simulink model "CNcs7"  (Simulink 6.2)
settings: Solver=ode4  SolverMode=SingleTasking  StartTime=0.0  StopTime=5  FixedStep=0.001  MaxStep=0.001  RelTol=1e-3  AbsTol=1e-3
undefined symbols (not defined in the file): alexlaw, bs_onoff, bs_scale, bsfsacrit, bsfsvcrit, cnsgain, fs_onoff, fs_scale, fsdelaycalc, ltdrk, phasicgain, pmcgain, pmctau2, pmctau3, saccrefract, saccsw, spgain, tonicgain, tvrD, tvrN, velnoise, velreconsw
libraries: simulink_extras x38, simulink x2
(part 2 of 5)

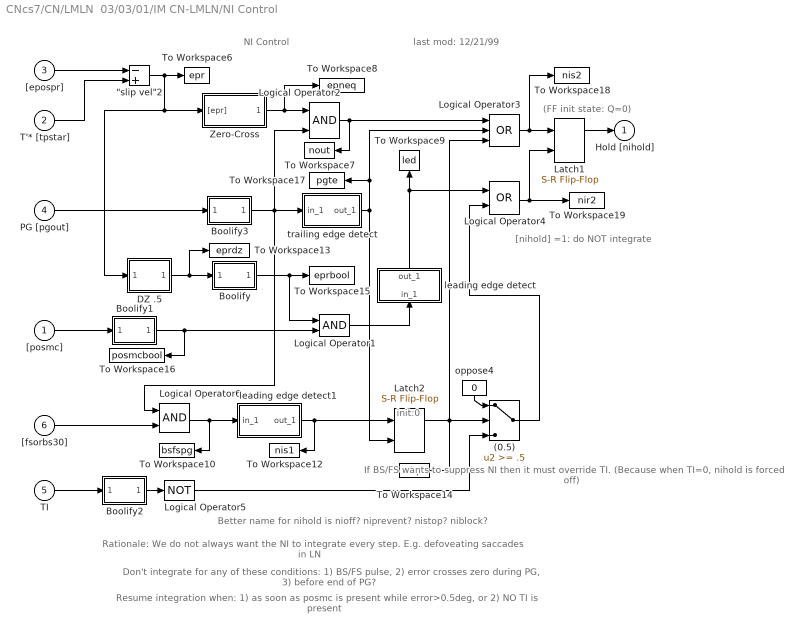
== system CNcs7/CN/LMLN  03/03/01/IM CN-LMLN/NI Control ==
  note: (FF init state: Q=0)
  note: NI Control
  note: If BS/FS wants to suppress NI
      | then it must override TI. (Because
      | when TI=0, nihold is forced off)
  note: last mod:
      | 12/21/99
  note: Rationale: We do not always want the NI to integrate every step. E.g. defoveating saccades in LN
  note: Don't integrate for any of these conditions: 1) BS/FS pulse, 2) error crosses zero during PG, 3) before end of PG?
  note: [nihold] =1: do NOT integrate
  note: init:0
  note: Better name for nihold is nioff? niprevent? nistop? niblock?
  note: Resume integration when: 1) as soon as posmc is present while error>0.5deg, or 2) NO TI is present
  "[posmc]" : Inport  Port=1  LatchInput=off
  T'* [tpstar] : Inport  Port=2  LatchInput=off
  "[epospr]" : Inport  Port=3  LatchInput=off
  PG [pgout] : Inport  Port=4  LatchInput=off
  TI : Inport  Port=5  LatchInput=off
  "[fsorbs30]" : Inport  Port=6  LatchInput=off
  "\"slip vel\"2" : Sum  Inputs=-+  SaturateOnIntegerOverflow=on  InputSameDT=on
  (0.5) : Switch  Threshold=.5  SaturateOnIntegerOverflow=on  InputSameDT=on
  Boolify : Subsystem
      mask Display: disp('Boolify')
  Boolify1 : Subsystem
      mask Display: disp('Boolify')
  Boolify2 : Subsystem
      mask Display: disp('Boolify')
  Boolify3 : Subsystem
      mask Display: disp('Boolify')
  DZ .5 : Subsystem
      mask Display: disp('Dead\nZone')
  Latch1 : simulink_extras/Flip Flops/S-R Flip-Flop  initial_condition=0
  Latch2 : simulink_extras/Flip Flops/S-R Flip-Flop  initial_condition=0
  Logical Operator1 : Logic
  Logical Operator2 : Logic
  Logical Operator3 : Logic  Operator=OR  Inputs=3
  Logical Operator4 : Logic  Operator=OR
  Logical Operator5 : Logic  Operator=NOT  Inputs=1
  Logical Operator6 : Logic
  To Workspace10 : ToWorkspace  VariableName=bsfspg  SaveFormat=Array
      settings: MaxDataPoints=10000
  To Workspace12 : ToWorkspace  VariableName=nis1  SaveFormat=Array
      settings: MaxDataPoints=10000
  To Workspace13 : ToWorkspace  VariableName=eprdz  SaveFormat=Array
      settings: MaxDataPoints=10000
  To Workspace14 : ToWorkspace  VariableName=niq1  SaveFormat=Array
      settings: MaxDataPoints=10000
  To Workspace15 : ToWorkspace  VariableName=eprbool  SaveFormat=Array
      settings: MaxDataPoints=10000
  To Workspace16 : ToWorkspace  VariableName=posmcbool  SaveFormat=Array
      settings: MaxDataPoints=10000
  To Workspace17 : ToWorkspace  VariableName=pgte  SaveFormat=Array
      settings: MaxDataPoints=10000
  To Workspace18 : ToWorkspace  VariableName=nis2  SaveFormat=Array
      settings: MaxDataPoints=10000
  To Workspace19 : ToWorkspace  VariableName=nir2  SaveFormat=Array
      settings: MaxDataPoints=10000
  To Workspace6 : ToWorkspace  VariableName=epr  SaveFormat=Array
      settings: MaxDataPoints=10000
  To Workspace7 : ToWorkspace  VariableName=nout  SaveFormat=Array
      settings: MaxDataPoints=10000
  To Workspace8 : ToWorkspace  VariableName=epneq  SaveFormat=Array
      settings: MaxDataPoints=10000
  To Workspace9 : ToWorkspace  VariableName=led  SaveFormat=Array
      settings: Orientation=up  MaxDataPoints=10000
  Zero-Cross : Subsystem
      mask Display: disp('Zero-Cross\nDetect')
  leading edge detect : Subsystem  Orientation=up
      mask Display: disp('Leading\nEdge Det')
  leading edge detect1 : Subsystem
      mask Display: disp('Leading\nEdge Det')
  oppose4 : Constant  Orientation=down  Value=0
  trailing edge detect : Subsystem
      mask Display: disp('Trailing\nEdge Det')
  Hold [nihold] : Outport
  wires:
  T'* [tpstar]/1 -> "\"slip vel\"2"/2
  PG [pgout]/1 -> Boolify3/1(In1)
  "\"slip vel\"2"/1 -> To Workspace6/1, DZ .5/1(in_1), Zero-Cross/1("[epr]")
  "[epospr]"/1 -> "\"slip vel\"2"/1
  Latch1/1 -> Hold [nihold]/1
  Logical Operator3/1 -> Latch1/1, To Workspace18/1
  Zero-Cross/1("[epneq]") -> Logical Operator2/1, To Workspace8/1
  Logical Operator1/1 -> leading edge detect/1(in_1)
  Logical Operator2/1 -> Logical Operator3/1, To Workspace7/1
  "[fsorbs30]"/1 -> Logical Operator6/2
  Logical Operator6/1 -> leading edge detect1/1(in_1), To Workspace10/1
  Latch2/1 -> Logical Operator3/3, (0.5)/2, To Workspace14/1
  oppose4/1 -> (0.5)/1
  Logical Operator5/1 -> (0.5)/3
  leading edge detect1/1(out_1) -> Latch2/1, To Workspace12/1
  Logical Operator4/1 -> Latch1/2, To Workspace19/1
  TI/1 -> Boolify2/1(In1)
  Boolify2/1(Out1) -> Logical Operator5/1
  leading edge detect/1(out_1) -> To Workspace9/1, Logical Operator4/1
  (0.5)/1 -> Logical Operator4/2
  Boolify3/1(Out1) -> Logical Operator6/1, trailing edge detect/1(in_1), Logical Operator2/2
  trailing edge detect/1(out_1) -> To Workspace17/1, Logical Operator3/2, Latch2/2
  Boolify/1(Out1) -> To Workspace15/1, Logical Operator1/1
  DZ .5/1(out_1) -> Boolify/1(In1), To Workspace13/1
  "[posmc]"/1 -> Boolify1/1(In1)
  Boolify1/1(Out1) -> To Workspace16/1, Logical Operator1/2

== system CNcs7/CN/LMLN  03/03/01/IM CN-LMLN/Sacc Blank ==
  note: Saccade and Post-Saccadic Drift Blanking
  note: (FF init state: Q=1)
  note: "Is RetVel Err increaing?"
  note: really an "enable"
      | signal?
  note: last mod:
      | 02/03/00
  note: [sbsac]  is initially ENABLED, and is DISABLED by  the leading edge of a saccade
      |  (after an 80ms delay).  70 ms later the timer REENABLES [sbsac]
      | (Because of the 80ms delay, actual time of reenable is150 ms after end of PG)
  note: Lower SR latch is SET by [sbsac] going high.  The switch will now pass information
      | about the change in velocity error (whether it is decreasing or increasing).
      | If it is increasing, [sbsp] is 1, and the beginning of this increase sets the switch so
      | that [sbsp] = [sbsac].  If the error is decreasing, then [sbsp] = 0, and should stay 0
      |  for as long as [velerr] is decreasing ***and hasn't crossed zero***
  note: Rationale: We do not want the model to look at the slow phase information that immediately
      | follows a saccade.   We want to disable both the saccadic and SP systems appropriately.
  note: Saccadic:
  note: SP:
  note: (init: Q=0)
  note: "non-decreasing"
  PG [pgout] : Inport  Port=1  LatchInput=off
  RetVelErr [velerr] : Inport  Port=2  LatchInput=off
  Abs1 : Abs  SaturateOnIntegerOverflow=on
  Latch1 : simulink_extras/Flip Flops/S-R Flip-Flop  initial_condition=1
  Latch2 : simulink_extras/Flip Flops/S-R Flip-Flop  initial_condition=0
  Relational Operator : RelationalOperator  InputSameDT=on
  Switch5 : Switch  Threshold=.5  SaturateOnIntegerOverflow=on  InputSameDT=on
  To Workspace10 : ToWorkspace  VariableName=sbred  SaveFormat=Array
      settings: MaxDataPoints=10000
  To Workspace11 : ToWorkspace  VariableName=sbpsred  SaveFormat=Array
      settings: MaxDataPoints=10000
  To Workspace18 : ToWorkspace  VariableName=pg80  SaveFormat=Array
      settings: MaxDataPoints=10000
  To Workspace8 : ToWorkspace  VariableName=sbpsd  SaveFormat=Array
      settings: MaxDataPoints=10000
  To Workspace9 : ToWorkspace  VariableName=sbcs  SaveFormat=Array
      settings: MaxDataPoints=10000
  Transport Delay1 : TransportDelay  DelayTime=0.080
      mask Display: disp('80ms')
  event timer1 : Subsystem
      mask Display: disp('Event\nTimer2')
  leading edge detect : Subsystem
      mask Display: disp('Leading\nEdge Det')
  loop breaker : Memory
  rising edge detect : Subsystem  Orientation=left
      mask Display: disp('Rising\nEdge Det')
  rising edge detect1 : Subsystem
      mask Display: disp('Rising\nEdge Det')
  timer value : Constant  Orientation=left  Value=.07
  SacBlnk [sbsac] : Outport
  SP S/H [sbsp] : Outport  Port=2
  wires:
  leading edge detect/1(out_1) -> Latch1/2
  event timer1/1(out_1) -> Latch1/1
  loop breaker/1 -> Relational Operator/2
  Abs1/1 -> loop breaker/1, Relational Operator/1
  Relational Operator/1 -> To Workspace8/1, rising edge detect/1(in_1), Switch5/1
  rising edge detect1/1(out_1) -> To Workspace10/1, Latch2/1
  Switch5/1 -> SP S/H [sbsp]/1
  RetVelErr [velerr]/1 -> Abs1/1
  rising edge detect/1(out_1) -> Latch2/2, To Workspace11/1
  Latch2/1 -> Switch5/2, To Workspace9/1
  PG [pgout]/1 -> Transport Delay1/1
  Transport Delay1/1 -> leading edge detect/1(in_1), event timer1/1(_PG), To Workspace18/1
  timer value/1 -> event timer1/2(_timer value (port))
  Latch1/1 -> SacBlnk [sbsac]/1, rising edge detect1/1(in_1), Switch5/3

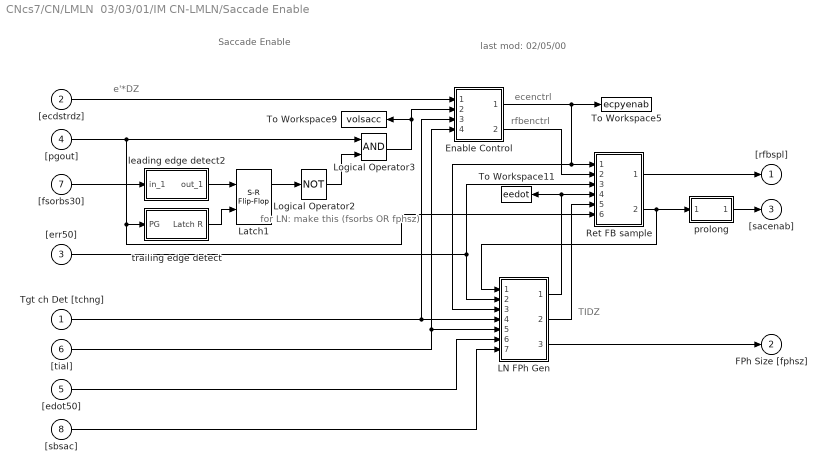
== system CNcs7/CN/LMLN  03/03/01/IM CN-LMLN/Saccade Enable ==
  note: Saccade Enable
  note: last mod:
      | 02/05/00
  note: rfbenctrl
  note: ecenctrl
  note: e'*DZ
  note: for LN: make this
      | (fsorbs OR fphsz)
  note: TIDZ
  Tgt ch Det [tchng] : Inport  Port=1  LatchInput=off
  "[ecdstrdz]" : Inport  Port=2  LatchInput=off
  "[err50]" : Inport  Port=3  LatchInput=off
  "[pgout]" : Inport  Port=4  LatchInput=off
  "[edot50]" : Inport  Port=5  LatchInput=off
  "[tial]" : Inport  Port=6  LatchInput=off
  "[fsorbs30]" : Inport  Port=7  LatchInput=off
  "[sbsac]" : Inport  Port=8  LatchInput=off
  Enable Control : Subsystem
      mask Display: disp('Enable\nControl')
  LN FPh Gen : Subsystem
      mask Display: disp('DFFPh\nGen')
  Latch1 : simulink_extras/Flip Flops/S-R Flip-Flop  initial_condition=0
  Logical Operator2 : Logic  Operator=NOT  Inputs=1
  Logical Operator3 : Logic
  Ret FB sample : Subsystem
      mask Display: disp('Ret FB\nEnab &\nSample')
  To Workspace11 : ToWorkspace  VariableName=eedot  SaveFormat=Array
      settings: MaxDataPoints=10000
  To Workspace5 : ToWorkspace  VariableName=ecpyenab  SaveFormat=Array
      settings: MaxDataPoints=10000
      mask Type: imsw1in
  To Workspace9 : ToWorkspace  VariableName=volsacc  SaveFormat=Array
      settings: MaxDataPoints=10000
      mask Type: imsw1in
  leading edge detect2 : Subsystem
      mask Display: disp('Leading\nEdge Det')
  prolong : Subsystem  mask{prolong=10}
      mask prompts: prolong "Prolong pulse by?  (msec)"
      mask Display: disp('prolong')
  trailing edge detect : Subsystem
      mask Display: disp('Trailing\nEdge Det')
  "[rfbspl]" : Outport
  FPh Size [fphsz] : Outport  Port=2
  "[sacenab]" : Outport  Port=3
  wires:
  "[pgout]"/1 -> Logical Operator3/1, trailing edge detect/1(PG), Ret FB sample/6("[volsacct]")
  Logical Operator2/1 -> Logical Operator3/2
  "[ecdstrdz]"/1 -> Enable Control/1(e'*DZ [ecdstrdz])
  Ret FB sample/1(RFB Spl [rfbspl]) -> "[rfbspl]"/1
  Tgt ch Det [tchng]/1 -> LN FPh Gen/4(TCD [tchng]), Enable Control/3(Tgt ch Det [tchng])
  "[sbsac]"/1 -> LN FPh Gen/7("[sbsac]")
  "[edot50]"/1 -> LN FPh Gen/6("[edot50]")
  "[tial]"/1 -> LN FPh Gen/5("[tial]"), Enable Control/4("[tial]")
  Enable Control/1(ECPY EnTmng [ecpyenab]) -> LN FPh Gen/3("[ecpyenab]"), Ret FB sample/1("[ecpyenab]"), To Workspace5/1
  "[err50]"/1 -> LN FPh Gen/2("[err50]"), Ret FB sample/3("[err50]")
  Enable Control/2(RetFB En&Spl) -> Ret FB sample/2("[rfbenctrl]")
  LN FPh Gen/2(TIDZ) -> Ret FB sample/5(TIDZ)
  LN FPh Gen/3(FPh Size [fphsz]) -> FPh Size [fphsz]/1
  Ret FB sample/2(RetFB Enable [sacenab]) -> prolong/1(value(in)), LN FPh Gen/1("[rfbenab]")
  prolong/1(value(out)) -> "[sacenab]"/1
  "[fsorbs30]"/1 -> leading edge detect2/1(in_1)
  leading edge detect2/1(out_1) -> Latch1/1
  Latch1/1 -> Logical Operator2/1
  trailing edge detect/1(Latch R) -> Latch1/2
  LN FPh Gen/1("[eedot]") -> Ret FB sample/4("[eedot]"), To Workspace11/1
  Logical Operator3/1 -> Enable Control/2(VolPG ( [pgout] &NOT fs or bs)), To Workspace9/1

== system CNcs7/CN/LMLN  03/03/01/IM CN-LMLN/Saccade Motor Commmand ==
  note: last mod:
      | 02/25/01
  note: Saccadic Motor Command
  note: If TCHNG occurs, BLOCK
      | BS/FS (and already prog vs?)
      | for 150 msec
  note: mod so that tchng NECESSARY
      | input to 'Vol Sacc Sw'
      | this way can not have vol sacc
      | w/o tgt change?
  note: If TCHNG occurs:
      | ALLOW vol sacc
  note: make sure that tchngOVR
      | lets _something_ pass,
      | since it operates switches
      | in two different locations...
  "[ecdstrdz]" : Inport  Port=1  LatchInput=off
  "[fphsz]" : Inport  Port=2  LatchInput=off
  "[sacenab]" : Inport  Port=3  LatchInput=off
  "[fsorbs30]" : Inport  Port=4  LatchInput=off
  "[fsbcmc30]" : Inport  Port=5  LatchInput=off
  Tgt ch Det [tchng] : Inport  Port=6  LatchInput=off
  "\"slip vel\"1" : Sum  SaturateOnIntegerOverflow=on  InputSameDT=on
  (0.5) : Switch  Threshold=.5  SaturateOnIntegerOverflow=on  InputSameDT=on
  0 : Constant  Orientation=left  Value=0
  Switch3 : Switch  Threshold=.5  SaturateOnIntegerOverflow=on  InputSameDT=on
  TCHNG Override : Subsystem
      mask Display: disp('TCHNG\nOverride')
  To Workspace12 : ToWorkspace  VariableName=fphmag  SaveFormat=Array
      settings: MaxDataPoints=10000
  To Workspace13 : ToWorkspace  VariableName=vsmc  SaveFormat=Array
      settings: MaxDataPoints=10000
  Voluntary Saccade Switch : Subsystem
      mask Display: disp('Vol\nSacc\nSw')
  timer value : Constant  Orientation=left  Value=0.15
  "[posmc]" : Outport
  wires:
  "[ecdstrdz]"/1 -> "\"slip vel\"1"/1
  "[fphsz]"/1 -> "\"slip vel\"1"/2
  "[sacenab]"/1 -> Voluntary Saccade Switch/2("[sacenab]")
  "[fsbcmc30]"/1 -> (0.5)/3
  "\"slip vel\"1"/1 -> Voluntary Saccade Switch/1("[fphmag]"), To Workspace12/1
  Voluntary Saccade Switch/1("[vsmc]") -> (0.5)/1, To Workspace13/1
  0/1 -> Switch3/3
  Switch3/1 -> "[posmc]"/1
  (0.5)/1 -> Switch3/1
  "[fsorbs30]"/1 -> Voluntary Saccade Switch/3("[fsorbs30]")
  Voluntary Saccade Switch/2(sacenab/0) -> (0.5)/2
  TCHNG Override/1(tchng sw) -> Switch3/2, Voluntary Saccade Switch/4(tchng enable)
  Tgt ch Det [tchng]/1 -> TCHNG Override/1("[tchng]")
  timer value/1 -> TCHNG Override/2(timer dur)

== system CNcs7/CN/LMLN  03/03/01/IM CN-LMLN/Sampled Error Reconstruction ==
  note: e'*
  note: Sampled Error Reconstruction
  note: last mod:
      | 02/22/01
  note: [svtpr] is approx = to the CNvel signal and is used for CN simulations; for normals, [svtpr]
      | should be = 0 and sppr50 would not be switched into the summer
  note: [sv+tial]*k is used for the LMLN model and needs to be automatically switched off
      | for normals or CN simulations
  "[tpstar]" : Inport  Port=1  LatchInput=off
  "[epospr]" : Inport  Port=2  LatchInput=off
  (sv+tial) k : Inport  Port=3  LatchInput=off
  "[svtpr]" : Inport  Port=4  LatchInput=off
  TI : Inport  Port=5  LatchInput=off
  (0.5) : Switch  Threshold=.5  SaturateOnIntegerOverflow=on  InputSameDT=on
  (Init input:0) : Memory
  Boolify : Subsystem
      mask Display: disp('Boolify')
  Boolify1 : Subsystem
      mask Display: disp('Boolify')
  DZ 0.3 : Subsystem
      mask Display: disp('DZ 0.3')
  Integrator : Integrator
  Product6 : Product  SaturateOnIntegerOverflow=on  RndMeth=Zero  InputSameDT=on
  Sum6 : Sum  Inputs=+---  SaturateOnIntegerOverflow=on  InputSameDT=on
  To Workspace10 : ToWorkspace  VariableName=epospr50  SaveFormat=Array
      settings: MaxDataPoints=10000
  To Workspace11 : ToWorkspace  VariableName=sppr50sw  SaveFormat=Array
      settings: MaxDataPoints=10000
  To Workspace7 : ToWorkspace  VariableName=ecdstr  SaveFormat=Array
      settings: MaxDataPoints=10000
  To Workspace8 : ToWorkspace  VariableName=sppr  SaveFormat=Array
      settings: MaxDataPoints=10000
  To Workspace9 : ToWorkspace  VariableName=sppr50  SaveFormat=Array
      settings: MaxDataPoints=10000
  Transport Delay10 : TransportDelay  DelayTime=.05
      mask Display: disp('50ms')
  Transport Delay9 : TransportDelay  DelayTime=.05
      mask Display: disp('50ms')
  oppose5 : Constant  Orientation=left  Value=0
  "[ecdstrdz] (excl nystag)" : Outport
  wires:
  Transport Delay9/1 -> Sum6/2, To Workspace10/1
  TI/1 -> Boolify1/1(In1)
  Boolify1/1(Out1) -> Product6/2
  (sv+tial) k/1 -> Product6/1
  Product6/1 -> Sum6/3
  DZ 0.3/1(out_1) -> "[ecdstrdz] (excl nystag)"/1
  Sum6/1 -> To Workspace7/1, DZ 0.3/1(in_1)
  oppose5/1 -> (0.5)/3
  Integrator/1 -> Transport Delay10/1, To Workspace8/1
  Transport Delay10/1 -> (0.5)/1, To Workspace9/1
  "[svtpr]"/1 -> Integrator/1, Boolify/1(In1)
  (0.5)/1 -> To Workspace11/1, Sum6/4
  Boolify/1(Out1) -> (0.5)/2
  "[epospr]"/1 -> Transport Delay9/1
  "[tpstar]"/1 -> (Init input:0)/1
  (Init input:0)/1 -> Sum6/1

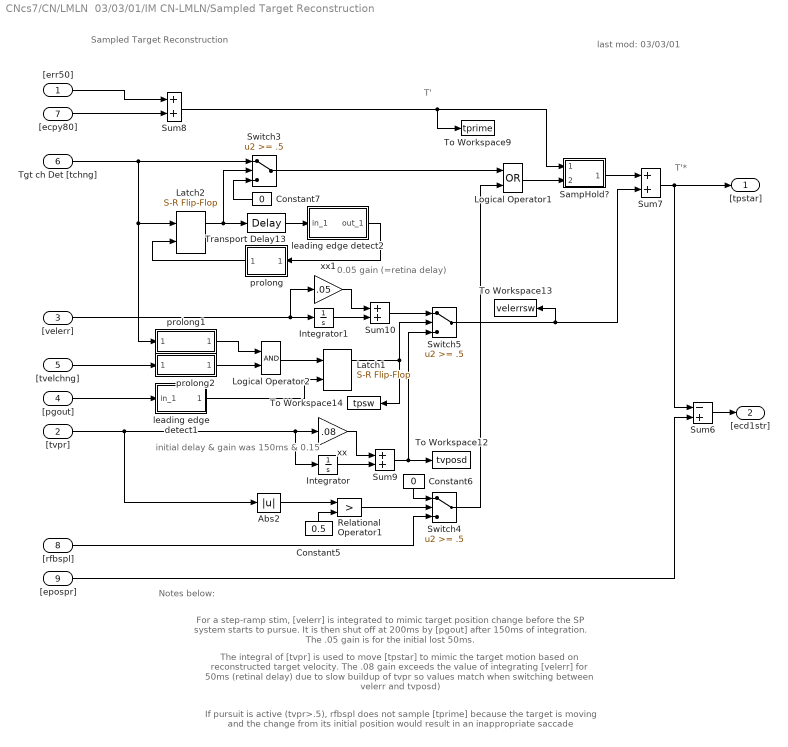
== system CNcs7/CN/LMLN  03/03/01/IM CN-LMLN/Sampled Target Reconstruction ==
  note: T'
  note: T'*
  note: Sampled Target Reconstruction
  note: last mod:
      | 03/03/01
  note: Notes below:
  note: If pursuit is active (tvpr>.5), rfbspl does not sample [tprime] because the target is moving and
      | the change from its initial position would result in an inappropriate saccade
  note: The integral of [tvpr] is used to move [tpstar] to mimic the target motion based on reconstructed target velocity. The .08 gain
      | exceeds the value of integrating [velerr] for 50ms (retinal delay) due to slow buildup of tvpr so values match
      | when switching between velerr and tvposd)
  note: For a step-ramp stim, [velerr] is integrated to mimic target position change before the SP system starts to pursue.
      |  It is then shut off at 200ms by [pgout] after 150ms of integration. The .05 gain is for the initial lost 50ms.
  note: initial delay & gain
      | was 150ms & 0.15
  note: 0.05 gain (=retina delay)
  "[err50]" : Inport  Port=1  LatchInput=off
  "[tvpr]" : Inport  Port=2  LatchInput=off
  "[velerr]" : Inport  Port=3  LatchInput=off
  "[pgout]" : Inport  Port=4  LatchInput=off
  "[tvelchng]" : Inport  Port=5  LatchInput=off
  Tgt ch Det [tchng] : Inport  Port=6  LatchInput=off
  "[ecpy80]" : Inport  Port=7  LatchInput=off
  "[rfbspl]" : Inport  Port=8  LatchInput=off
  "[epospr]" : Inport  Port=9  LatchInput=off
  Abs2 : Abs  SaturateOnIntegerOverflow=on
  Constant5 : Constant  Orientation=up  Value=0.5
  Constant6 : Constant  Orientation=down  Value=0
  Constant7 : Constant  Orientation=left  Value=0
  Integrator : Integrator
  Integrator1 : Integrator
  Latch1 : simulink_extras/Flip Flops/S-R Flip-Flop  initial_condition=0
  Latch2 : simulink_extras/Flip Flops/S-R Flip-Flop  initial_condition=0
  Logical Operator1 : Logic  Operator=OR
  Logical Operator2 : Logic
  Relational Operator1 : RelationalOperator  Operator=>  InputSameDT=on
  SampHold? : Subsystem
      mask Display: disp('S=H\nH=L')
  Sum{7..10} (4 alike) : Sum  SaturateOnIntegerOverflow=on  InputSameDT=on
  Sum6 : Sum  Inputs=-+  SaturateOnIntegerOverflow=on  InputSameDT=on
  Switch3 : Switch  Threshold=.5  SaturateOnIntegerOverflow=on  InputSameDT=on
  Switch4 : Switch  Threshold=.5  SaturateOnIntegerOverflow=on  InputSameDT=on
  Switch5 : Switch  Threshold=.5  SaturateOnIntegerOverflow=on  InputSameDT=on
  To Workspace12 : ToWorkspace  VariableName=tvposd  SaveFormat=Array
      settings: MaxDataPoints=10000
  To Workspace13 : ToWorkspace  VariableName=velerrsw  SaveFormat=Array
      settings: MaxDataPoints=10000
  To Workspace14 : ToWorkspace  VariableName=tpsw  SaveFormat=Array
      settings: MaxDataPoints=10000
  To Workspace9 : ToWorkspace  VariableName=tprime  SaveFormat=Array
      settings: MaxDataPoints=10000
  Transport Delay13 : TransportDelay  DelayTime=.05
      mask Display: disp('50ms')
  leading edge detect1 : Subsystem
      mask Display: disp('Leading\nEdge Det')
  leading edge detect2 : Subsystem
      mask Display: disp('Leading\nEdge Det')
  prolong : Subsystem  Orientation=left  mask{prolong=150}
      mask prompts: prolong "Prolong pulse by?  (msec)"
      mask Display: disp('150ms\nprolong')
  prolong1 : Subsystem  mask{prolong=5}
      mask prompts: prolong "Prolong pulse by?  (msec)"
      mask Display: disp('5ms prolong')
  prolong2 : Subsystem  mask{prolong=5}
      mask prompts: prolong "Prolong pulse by?  (msec)"
      mask Display: disp('5ms prolong')
  xx : Gain  Gain=.08  SaturateOnIntegerOverflow=on
  xx1 : Gain  Gain=.05  SaturateOnIntegerOverflow=on
  "[tpstar]" : Outport
  "[ecd1str]" : Outport  Port=2
  wires:
  Sum8/1 -> To Workspace9/1, SampHold?/1(Input)
  "[ecpy80]"/1 -> Sum8/2
  "[err50]"/1 -> Sum8/1
  Sum6/1 -> "[ecd1str]"/1
  Switch5/1 -> To Workspace13/1, Sum7/2
  prolong1/1(value(out)) -> Logical Operator2/1
  Tgt ch Det [tchng]/1 -> Switch3/1, Latch2/1, prolong1/1(value(in))
  Logical Operator1/1 -> SampHold?/2(S/H?)
  Sum7/1 -> "[tpstar]"/1, Sum6/1
  SampHold?/1(output) -> Sum7/1
  Switch3/1 -> Logical Operator1/1
  Constant7/1 -> Switch3/3
  Latch2/1 -> Switch3/2, Transport Delay13/1
  Transport Delay13/1 -> leading edge detect2/1(in_1)
  leading edge detect2/1(out_1) -> prolong/1(value(in))
  prolong/1(value(out)) -> Latch2/2
  Sum10/1 -> Switch5/1
  Integrator1/1 -> Sum10/2
  xx1/1 -> Sum10/1
  Abs2/1 -> Relational Operator1/1
  Constant6/1 -> Switch4/1
  "[epospr]"/1 -> Sum6/2
  Constant5/1 -> Relational Operator1/2
  Relational Operator1/1 -> Switch4/2
  "[rfbspl]"/1 -> Switch4/3
  Integrator/1 -> Sum9/2
  xx/1 -> Sum9/1
  "[tvpr]"/1 -> Abs2/1, xx/1, Integrator/1
  Sum9/1 -> To Workspace12/1, Switch5/3
  Switch4/1 -> Logical Operator1/2
  leading edge detect1/1(out_1) -> Latch1/2
  "[pgout]"/1 -> leading edge detect1/1(in_1)
  Logical Operator2/1 -> Latch1/1
  "[tvelchng]"/1 -> prolong2/1(value(in))
  prolong2/1(value(out)) -> Logical Operator2/2
  Latch1/1 -> Switch5/2, To Workspace14/1
  "[velerr]"/1 -> Integrator1/1, xx1/1

== system CNcs7/CN/LMLN  03/03/01/IM CN-LMLN/Slip Velocity Reconstruction ==
  note: last mod:
      | 02/05/00
  note: Slip Velocity Reconstruction
  "[tial]" : Inport  Port=1  LatchInput=off
  "[evelpr]" : Inport  Port=2  LatchInput=off
  "[tvpr]" : Inport  Port=3  LatchInput=off
  " 1" : Sum  Inputs=-+  SaturateOnIntegerOverflow=on  InputSameDT=on
  "\"slip vel\"" : Sum  Inputs=-+  SaturateOnIntegerOverflow=on  InputSameDT=on
  Sum9 : Sum  SaturateOnIntegerOverflow=on  InputSameDT=on
  Transport Delay12 : TransportDelay  DelayTime=.05
      mask Display: disp('50ms')
  spgain (Default: 0.95) : Gain  Gain=spgain  SaturateOnIntegerOverflow=on
  sv+tial : Sum  SaturateOnIntegerOverflow=on  InputSameDT=on
  xx : Gain  Gain=.15  SaturateOnIntegerOverflow=on
  Vel->Pos : Outport
  "[svtpr]" : Outport  Port=2
  "'slip vel\" [svpr]" : Outport  Port=3
  "[tialsp]" : Outport  Port=4
  wires:
  xx/1 -> Vel->Pos/1
  Sum9/1 -> "[tialsp]"/1
  sv+tial/1 -> xx/1
  "[tial]"/1 -> sv+tial/1, Sum9/1
  "\"slip vel\""/1 -> sv+tial/2, "'slip vel\" [svpr]"/1
  "[evelpr]"/1 -> Sum9/2, "\"slip vel\""/1, " 1"/1
  spgain (Default: 0.95)/1 -> " 1"/2
  " 1"/1 -> "[svtpr]"/1
  "[tvpr]"/1 -> Transport Delay12/1
  Transport Delay12/1 -> "\"slip vel\""/2, spgain (Default: 0.95)/1

== system CNcs7/CN/LMLN  03/03/01/IM CN-LMLN/Target Change Detection ==
  note: Target Change Detection
  note: Detects T change >1 deg any time
  RetErr Vel [edot50] : Inport  Port=1  LatchInput=off
  "[tvpr]" : Inport  Port=2  LatchInput=off
  Abs2 : Abs  SaturateOnIntegerOverflow=on
  Abs3 : Abs  SaturateOnIntegerOverflow=on
  Constant : Constant  Value=0
  Constant5 : Constant  Orientation=up  Value=950
  Constant6 : Constant  Orientation=up  Value=950
  Derivative : Derivative
      mask Display: disp('s')
  Relational Operator : RelationalOperator  InputSameDT=on
  Relational Operator1 : RelationalOperator  InputSameDT=on
  Terminator : Terminator
  prolong : Subsystem  mask{prolong=5}
      mask prompts: prolong "Prolong pulse by?  (msec)"
      mask Display: disp('prolong')
  Trgt Chng [tchng] : Outport
  Tvel Chng [tvelchng] : Outport  Port=2
  wires:
  RetErr Vel [edot50]/1 -> Abs2/1
  Constant5/1 -> Relational Operator/2
  Abs2/1 -> Relational Operator/1
  Constant6/1 -> Relational Operator1/2
  Abs3/1 -> Relational Operator1/1
  "[tvpr]"/1 -> Derivative/1
  Derivative/1 -> Abs3/1
  Relational Operator/1 -> Trgt Chng [tchng]/1
  Relational Operator1/1 -> Tvel Chng [tvelchng]/1
  prolong/1(value(out)) -> Terminator/1
  Constant/1 -> prolong/1(value(in))

== system CNcs7/CN/LMLN  03/03/01/IM CN-LMLN/Target Velocity Reconstruction1 ==
  note: last mod:
      | 02/22/00
  note: Target Velocity Reconstruction
  note: This block has been simplified by removing the first stage of S&H (triggered by [sbsac]) as it is no longer necessary,
      | since we no longer use [dspvel] (a slow phase correction signal) which required us to blank the combination of it
      | and [imvel] (formerly [imsp]) in a futile attempt to properly reconstruct target velocity.  This modification has been tested
      | for PPfs and Pfs waveforms using step, ramp and step-ramp stimuli, and compared to the previous, more complex
      | version.  The results were identical in every case.
  "[imvel]" : Inport  Port=1  LatchInput=off
  "[sbsp]" : Inport  Port=2  LatchInput=off
  "[edot50]" : Inport  Port=3  LatchInput=off
  DZ 0.5 : Subsystem
      mask Display: disp('Dead\nZone')
  Lim 100 : Subsystem
      mask Display: disp('Limiter')
  P1 : Gain  SaturateOnIntegerOverflow=on
  SampHold?4 : Subsystem
      mask Display: disp('S=H\nH=L')
  Sum7 : Sum  SaturateOnIntegerOverflow=on  InputSameDT=on
  To Workspace23 : ToWorkspace  VariableName=spsh  SaveFormat=Array
      settings: MaxDataPoints=10000
  To Workspace24 : ToWorkspace  VariableName=splpf  SaveFormat=Array
      settings: MaxDataPoints=10000
  To Workspace28 : ToWorkspace  VariableName=tvlpr  SaveFormat=Array
      settings: MaxDataPoints=10000
  Transfer Fcn4 : TransferFcn  Numerator=[tvrN]  Denominator=[tvrD tvrN]
  dead zone : Constant  Orientation=up
  "[velerr]" : Outport
  "[tvpr]" : Outport  Port=2
  wires:
  dead zone/1 -> DZ 0.5/2(in_2)
  DZ 0.5/1(out_1) -> P1/1
  P1/1 -> "[tvpr]"/1
  Sum7/1 -> SampHold?4/1(Input), To Workspace28/1
  Transfer Fcn4/1 -> DZ 0.5/1(in_1), To Workspace24/1
  SampHold?4/1(output) -> To Workspace23/1, Transfer Fcn4/1
  "[sbsp]"/1 -> SampHold?4/2(S/H?)
  "[imvel]"/1 -> Sum7/2
  "[edot50]"/1 -> Lim 100/1(in_1)
  Lim 100/1(out_1) -> "[velerr]"/1, Sum7/1

== system CNcs7/CN/LMLN  03/03/01/IM CN-LMLN/setmdlp ==

== system CNcs7/CN/LMLN  03/03/01/NI Leaky/NI Real ==
  in_1 : Inport  Port=1  LatchInput=off
  Gain : Gain  Gain=25  SaturateOnIntegerOverflow=on
  Gain1 : Gain  Orientation=left  SaturateOnIntegerOverflow=on
  Sum : Sum  SaturateOnIntegerOverflow=on  InputSameDT=on
  Transfer Fcn : TransferFcn  Numerator=[1/25]  Denominator=[1 1/25]
  out_1 : Outport
  wires:
  Transfer Fcn/1 -> Gain1/1, out_1/1
  Gain1/1 -> Sum/1
  Sum/1 -> Transfer Fcn/1
  Gain/1 -> Sum/2
  in_1/1 -> Gain/1

== system CNcs7/CN/LMLN  03/03/01/OMN2/SampHold? ==
  note: When "S/H?" is LOW, then "Input" is switched directly to the
      | output ("sample").  When "S/H?" is HIGH, the current output is
      | maintained ("hold").
  Input : Inport  Port=1  LatchInput=off
  S/H? : Inport  Port=2  LatchInput=off
  Memory : Memory  Orientation=left
  Sign : Signum
  Switch2 : Switch  Threshold=0.5  SaturateOnIntegerOverflow=on  InputSameDT=on
  output : Outport
  wires:
  Switch2/1 -> Memory/1, output/1
  Memory/1 -> Switch2/1
  Input/1 -> Switch2/3
  Sign/1 -> Switch2/2
  S/H?/1 -> Sign/1

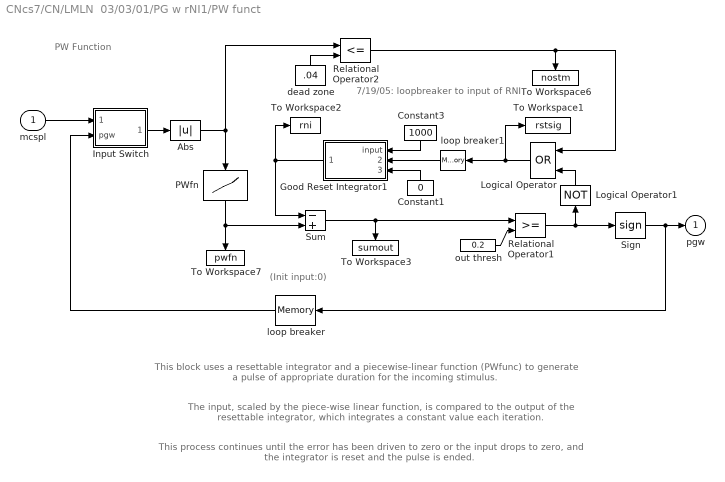
== system CNcs7/CN/LMLN  03/03/01/PG w rNI1/PW funct ==
  note: This process continues until the error has been driven to zero or the input drops to zero,
      | and the integrator is reset and the pulse is ended.
  note: The input, scaled by the piece-wise linear function, is compared to the output of the
      | resettable integrator, which integrates a constant value each iteration.
  note: This block uses a resettable integrator and a piecewise-linear function (PWfunc) to generate
      | a pulse of appropriate duration for the incoming stimulus.
  note: (Init input:0)
  note: PW Function
  note: 7/19/05: loopbreaker to input of RNI
  mcspl : Inport  Port=1  LatchInput=off
  Abs : Abs  SaturateOnIntegerOverflow=on
  Constant1 : Constant  Orientation=up  Value=0
  Constant3 : Constant  Orientation=down  Value=1000
  Good Reset Integrator1 : Subsystem  Orientation=left
      mask Display: disp('Resettable\nNI')
  Input Switch : Subsystem
      mask Display: disp('Input\nSwitch')
  Logical Operator : Logic  Orientation=left  Operator=OR
  Logical Operator1 : Logic  Orientation=up  Operator=NOT  Inputs=1
  PWfn : Lookup  Orientation=down  InputValues=[ 0, 0.1:5, 5:10, 10:50 ]  OutputValues="[ 0, (0.1:5)*0+15,  (5:10)*1+10,  (10:50)*2]"  SaturateOnIntegerOverflow=on
  Relational Operator1 : RelationalOperator  InputSameDT=on
  Relational Operator2 : RelationalOperator  Operator=<=  InputSameDT=on
  Sign : Signum
  Sum : Sum  Inputs=-+  SaturateOnIntegerOverflow=on  InputSameDT=on
  To Workspace1 : ToWorkspace  VariableName=rstsig  SaveFormat=Array
      settings: MaxDataPoints=10000
  To Workspace2 : ToWorkspace  VariableName=rni  SaveFormat=Array
      settings: MaxDataPoints=10000
  To Workspace3 : ToWorkspace  VariableName=sumout  SaveFormat=Array
      settings: Orientation=down  MaxDataPoints=10000
  To Workspace6 : ToWorkspace  VariableName=nostm  SaveFormat=Array
      settings: Orientation=down  MaxDataPoints=10000
  To Workspace7 : ToWorkspace  VariableName=pwfn  SaveFormat=Array
      settings: Orientation=down  MaxDataPoints=10000
  dead zone : Constant  Orientation=up  Value=.04
  loop breaker : Memory  Orientation=left
  loop breaker1 : Memory  Orientation=left
  out thresh : Constant  Value=0.2
  pgw : Outport
  wires:
  Logical Operator1/1 -> Logical Operator/2
  Relational Operator1/1 -> Logical Operator1/1, Sign/1
  Constant3/1 -> Good Reset Integrator1/1(input)
  Constant1/1 -> Good Reset Integrator1/3(initial condition)
  out thresh/1 -> Relational Operator1/2
  dead zone/1 -> Relational Operator2/2
  Relational Operator2/1 -> To Workspace6/1, Logical Operator/1
  Good Reset Integrator1/1(out_1) -> To Workspace2/1, Sum/1
  Logical Operator/1 -> To Workspace1/1, loop breaker1/1
  Sum/1 -> Relational Operator1/1, To Workspace3/1
  Input Switch/1(mcsw) -> Abs/1
  mcspl/1 -> Input Switch/1(mcspl)
  loop breaker/1 -> Input Switch/2(pgw)
  Sign/1 -> pgw/1, loop breaker/1
  PWfn/1 -> To Workspace7/1, Sum/2
  Abs/1 -> PWfn/1, Relational Operator2/1
  loop breaker1/1 -> Good Reset Integrator1/2(reset?)

== system CNcs7/CN/LMLN  03/03/01/PG w rNI1/RefLatch (Default = 50ms) ==
  note: It's a cheap trick, but it seems to work:
  note: The falling edge" block's output becomes DISABLED upon
      | detection of the END of the input pulse, and remains
      | so until the refractory period of rp milliseconds has elapsed.
  note: By ANDing these outputs, we get a signal that is DISABLED
      | starting with the beginning of the input pulse, and remains so until
      | rp milliseconds after the termination of the pulse.
  note: The "NOT" gate outputs a DISABLE signal whenever there is any
      | input, so that there can be no response.
  in_1 : Inport  Port=1  LatchInput=off
  Abs : Abs  SaturateOnIntegerOverflow=on
  Logical Operator : Logic
  Logical Operator1 : Logic  Operator=NOT  Inputs=1
  trailing edge : Subsystem
      mask Display: disp('Refract\nLatch (te)')
  out_1 : Outport
  wires:
  Logical Operator/1 -> out_1/1
  Logical Operator1/1 -> Logical Operator/1
  trailing edge/1(out_1) -> Logical Operator/2
  Abs/1 -> Logical Operator1/1, trailing edge/1(in_1)
  in_1/1 -> Abs/1

== system CNcs7/CN/LMLN  03/03/01/PG w rNI1/SampHold?1 ==
  note: When "S/H?" is HIGH, then "Input" is switched directly to the
      | output ("sample").  When "S/H?" is LOW, the current output is
      | maintained ("hold").
  Input : Inport  Port=1  LatchInput=off
  S/H? : Inport  Port=2  LatchInput=off
  Memory : Memory  Orientation=left
  Sign : Signum
  Switch2 : Switch  Threshold=0.5  SaturateOnIntegerOverflow=on  InputSameDT=on
  output : Outport
  wires:
  S/H?/1 -> Sign/1
  Sign/1 -> Switch2/2
  Input/1 -> Switch2/1
  Switch2/1 -> output/1, Memory/1
  Memory/1 -> Switch2/3

== system CNcs7/CN/LMLN  03/03/01/Fixation/30 /SampHold?2 ==
  note: When "S/H?" is LOW, then "Input" is switched directly to the
      | output ("sample").  When "S/H?" is HIGH, the current output is
      | maintained ("hold").
  Input : Inport  Port=1  LatchInput=off
  S/H? : Inport  Port=2  LatchInput=off
  Memory : Memory  Orientation=left
  Sign : Signum
  Switch2 : Switch  Threshold=0.5  SaturateOnIntegerOverflow=on  InputSameDT=on
  output : Outport
  wires:
  S/H?/1 -> Sign/1
  Sign/1 -> Switch2/2
  Input/1 -> Switch2/3
  Switch2/1 -> Memory/1, output/1
  Memory/1 -> Switch2/1

== system CNcs7/CN/LMLN  03/03/01/Fixation/30 /leading edge detect ==
  note: leading edge detection
  in_1 : Inport  Port=1  LatchInput=off
  Abs : Abs  SaturateOnIntegerOverflow=on
  Derivative : Derivative
  Relational Operator : RelationalOperator  Operator===  InputSameDT=on
  Sign : Signum
  Threshold 1 : Constant
  out_1 : Outport
  wires:
  in_1/1 -> Abs/1
  Relational Operator/1 -> out_1/1
  Threshold 1/1 -> Relational Operator/2
  Sign/1 -> Relational Operator/1
  Derivative/1 -> Sign/1
  Abs/1 -> Derivative/1

== system CNcs7/CN/LMLN  03/03/01/Fixation/30 /trailing edge detect ==
  note: It is also possible to remove the SIGNUM function
      | and the '==', and replace them with a simple
      | switch with a threshold of (say) 150 or so.
  note: trailing edge detection
  in_1 : Inport  Port=1  LatchInput=off
  Abs : Abs  SaturateOnIntegerOverflow=on
  Derivative : Derivative
  Relational Operator : RelationalOperator  Operator===  InputSameDT=on
  Sign : Signum
  Threshold 1 : Constant  Value=-1
  out_1 : Outport
  wires:
  Abs/1 -> Derivative/1
  Derivative/1 -> Sign/1
  Sign/1 -> Relational Operator/1
  Threshold 1/1 -> Relational Operator/2
  Relational Operator/1 -> out_1/1
  in_1/1 -> Abs/1

== system CNcs7/CN/LMLN  03/03/01/IM CN-LMLN/Alexander's law/Boolify ==
  TI : Inport  Port=1  LatchInput=off
  Abs2 : Abs  SaturateOnIntegerOverflow=on
  direction1 : Signum
  Switch Control : Outport
  wires:
  Abs2/1 -> direction1/1
  TI/1 -> Abs2/1
  direction1/1 -> Switch Control/1

== system CNcs7/CN/LMLN  03/03/01/IM CN-LMLN/BS/FS Logic/BS Enable1 ==
  note: BS Enable
  note: This block allows a BS for up to xx ms (set by "timer value")
      | after the acceleration criterion is met (i.e., drops below threshold)
  note: last mod:
      | 12/08/99
  note: (Default = 40deg/sec^2)
  bsprod : Inport  Port=1  LatchInput=off
  "[evelpr]" : Inport  Port=2  LatchInput=off
  Abs1 : Abs  SaturateOnIntegerOverflow=on
  BS Timing : Subsystem
      mask Display: disp('BS\nEnable\nTiming')
  Derivative : Derivative
      mask Display: disp('s')
  Relational Operator3 : RelationalOperator  Operator=<=  InputSameDT=on
  Switch4 : Switch  Threshold=.5  SaturateOnIntegerOverflow=on  InputSameDT=on
  To Workspace14 : ToWorkspace  VariableName=bscmpr  SaveFormat=Array
      settings: MaxDataPoints=10000
      mask Type: imsw1in
  To Workspace15 : ToWorkspace  VariableName=bsenab  SaveFormat=Array
      settings: MaxDataPoints=10000
      mask Type: imsw1in
  To Workspace16 : ToWorkspace  VariableName=bsaccel1  SaveFormat=Array
      settings: MaxDataPoints=10000
      mask Type: imsw1in
  "accel. thresh " : Constant  Orientation=up  Value=bsfsacrit
  off : Constant  Orientation=up  Value=0
  timer value : Constant  Orientation=up  Value=0.01
  "[bsmc]" : Outport
  wires:
  Relational Operator3/1 -> To Workspace14/1, BS Timing/1(From  <= [cmpr])
  Derivative/1 -> To Workspace16/1, Abs1/1
  Abs1/1 -> Relational Operator3/1
  BS Timing/1("[bsenab]") -> To Workspace15/1, Switch4/2
  "[evelpr]"/1 -> Derivative/1
  off/1 -> Switch4/3
  bsprod/1 -> Switch4/1
  Switch4/1 -> "[bsmc]"/1
  timer value/1 -> BS Timing/2(timer dur)
  "accel. thresh "/1 -> Relational Operator3/2

== system CNcs7/CN/LMLN  03/03/01/IM CN-LMLN/BS/FS Logic/FS Enable ==
  note: This block allows a FS for up to xx ms (set by "timer value")
      | after the acceleration criterion is met (i.e., drops below threshold)
  note: FS Enable
  note: last mod:
      | 12/08/99
  note: (Default = 40deg/sec^2)
  fsprod : Inport  Port=1  LatchInput=off
  "[evelpr]" : Inport  Port=2  LatchInput=off
  Abs1 : Abs  SaturateOnIntegerOverflow=on
  Derivative : Derivative
      mask Display: disp('s')
  FS Timing : Subsystem
      mask Display: disp('FS\nEnable\nTiming')
  Relational Operator3 : RelationalOperator  Operator=<=  InputSameDT=on
  SampHold?1 : Subsystem
      mask Display: disp('S=L\nH=H')
  Switch4 : Switch  Threshold=.5  SaturateOnIntegerOverflow=on  InputSameDT=on
  To Workspace14 : ToWorkspace  VariableName=fscmpr  SaveFormat=Array
      settings: MaxDataPoints=10000
      mask Type: imsw1in
  To Workspace15 : ToWorkspace  VariableName=fsenab  SaveFormat=Array
      settings: MaxDataPoints=10000
      mask Type: imsw1in
  To Workspace16 : ToWorkspace  VariableName=fsaccel1  SaveFormat=Array
      settings: MaxDataPoints=10000
      mask Type: imsw1in
  accel. thresh : Constant  Orientation=up  Value=bsfsacrit
  off : Constant  Orientation=up  Value=0
  timer value : Constant  Orientation=up  Value=0.01
  "[fsmc]" : Outport
  wires:
  timer value/1 -> FS Timing/2(timer dur)
  accel. thresh/1 -> Relational Operator3/2
  "[evelpr]"/1 -> Derivative/1
  FS Timing/1("[fsenab]") -> To Workspace15/1, SampHold?1/2(S/H?), Switch4/2
  Abs1/1 -> Relational Operator3/1
  Derivative/1 -> Abs1/1, To Workspace16/1
  Relational Operator3/1 -> FS Timing/1(From  <= [cmpr]), To Workspace14/1
  fsprod/1 -> SampHold?1/1(Input)
  Switch4/1 -> "[fsmc]"/1
  off/1 -> Switch4/3
  SampHold?1/1(output) -> Switch4/1

== system CNcs7/CN/LMLN  03/03/01/IM CN-LMLN/BS/FS Logic/FS or BS? ==
  note: The position error is compared to its value 3 milliseconds earlier.
      | If the error is _increasing_, we want to make a braking
      | saccade to oppose the runaway.
  note: If the position error is _decreasing_, then the eye is approaching the
      | target, and we would like to generate a foveating saccade, since
      | this is our best time to consider capturing the target.
  note: FS or BS?
  note: *****
  note: use diff & filter?
  pos error [ecd1str] : Inport  Port=1  LatchInput=off
  pgout : Inport  Port=2  LatchInput=off
  Abs : Abs  SaturateOnIntegerOverflow=on
  Boolify : Subsystem
      mask Display: disp('Boolify')
  Relational Operator : RelationalOperator  Operator=>  InputSameDT=on
  Relational Operator1 : RelationalOperator  InputSameDT=on
  SampHold?1 : Subsystem
      mask Display: disp('S&H\n(S=L)\n(H=H)')
  Transport Delay1 : TransportDelay  DelayTime=.002
      mask Display: disp('2ms')
  Transport Delay2 : TransportDelay  DelayTime=.001
      mask Display: disp('2ms')
  BS=1 FS=0 : Outport
  wires:
  Transport Delay1/1 -> Relational Operator/2
  pos error [ecd1str]/1 -> Abs/1
  Abs/1 -> Relational Operator/1, Transport Delay1/1
  pgout/1 -> Boolify/1(In1)
  Relational Operator/1 -> SampHold?1/1(Input)
  SampHold?1/1(output) -> BS=1 FS=0/1
  Boolify/1(Out1) -> SampHold?1/2(S/H?)

== system CNcs7/CN/LMLN  03/03/01/IM CN-LMLN/BS/FS Logic/TCHNG Override ==
  note: (FF init state: Q=1)
  note: * Leading Edge of input ENABLEs output
  note: Operation:
  note: *FS Enabling is initially DISABLED
  note: * Output of TIMER circuit DISABLES output
  note: TCHNG Override
  "[tchng]" : Inport  Port=1  LatchInput=off
  timer dur : Inport  Orientation=up  Port=2  LatchInput=off
  Latch1 : simulink_extras/Flip Flops/S-R Flip-Flop  initial_condition=1
  To Workspace13 : ToWorkspace  VariableName=tchngovr  SaveFormat=Array
      settings: Orientation=down  MaxDataPoints=10000
  event timer2 : Subsystem
      mask Display: disp('Event\nTimer2')
  leading edge detect : Subsystem
      mask Display: disp('Leading\nEdge Det')
  tchng sw : Outport
  wires:
  "[tchng]"/1 -> leading edge detect/1(in_1), event timer2/1(_PG)
  timer dur/1 -> event timer2/2(_timer value (port))
  event timer2/1(out_1) -> Latch1/1
  leading edge detect/1(out_1) -> Latch1/2
  Latch1/1 -> tchng sw/1, To Workspace13/1

== system CNcs7/CN/LMLN  03/03/01/IM CN-LMLN/BS/FS Logic/prolong ==
  note: init = 0
  note: init = 0
  note: 11/22/99
  note: The start of the input pulse causes the value on input 1 to be held starting when the leading
      | edge occurs, and this value remains latched until 'delay' seconds after the pulse ends (trailing edge).
  note: The one integration step delay before the S&H block's S/H (bottom) input insures
      | that the input value to be latched is available to theS&H block's top input
      | before the S&H block tries to 'hold'.
  note: Stretch the duration of an input pulse, latching it at its value at pulse onset.
  note: init Q = 0
  value(in) : Inport  Port=1  LatchInput=off
  " x/1000" : Constant  Orientation=up  Value=0.001
  Latch1 : simulink_extras/Flip Flops/S-R Flip-Flop  initial_condition=0
  Product : Product  SaturateOnIntegerOverflow=on  RndMeth=Zero  InputSameDT=on
  SampHold?2 : Subsystem
      mask Display: disp('S=L\nH=H')
  Variable Transport Delay : VariableTransportDelay  MaximumDelay=10  MaximumPoints=5120
  leading edge detect : Subsystem
      mask Display: disp('Leading\nEdge Det')
  loop breaker2 : Memory
  stretch : Constant  Value=prolong
  trailing edge detect : Subsystem
      mask Display: disp('Trailing\nEdge Det')
  value(out) : Outport
  wires:
  " x/1000"/1 -> Product/2
  Product/1 -> Variable Transport Delay/2
  stretch/1 -> Product/1
  loop breaker2/1 -> SampHold?2/2(S/H?)
  SampHold?2/1(output) -> value(out)/1
  Latch1/1 -> loop breaker2/1
  leading edge detect/1(out_1) -> Latch1/1
  trailing edge detect/1(out_1) -> Variable Transport Delay/1
  Variable Transport Delay/1 -> Latch1/2
  value(in)/1 -> SampHold?2/1(Input), trailing edge detect/1(in_1), leading edge detect/1(in_1)

== system CNcs7/CN/LMLN  03/03/01/IM CN-LMLN/MdlPlnt+/OMN2 ==
  note: OMN
  note: Note that the OMN properly combines the pulse with the output of the NI, by latching
      | that output to its value at the moment the pulse appears.
  note: Operation: when [pgout] is active it activates the switch, passing the
      | upper input through to the output.  When the pulse is over, the switch changes,
      | allowing the lower input (from the NI) to pass.
  note: This block behaves like the ocular motor neurons,combining a phasic pulse (from PG)
      | with the tonic step produced by integration of the step, yielding a Pulse-Step
      | to drive the plant.
  "[epossp]" : Inport  Port=1  LatchInput=off
  "[pgout]" : Inport  Port=2  LatchInput=off
  Abs : Abs  SaturateOnIntegerOverflow=on
  Gain _ : Gain  Gain=1.0  SaturateOnIntegerOverflow=on
  SampHold? : Subsystem
      mask Display: disp('S=L\nH=H')
  Sign : Signum
  Sum : Sum  SaturateOnIntegerOverflow=on  InputSameDT=on
  Switch : Switch  Threshold=.5  SaturateOnIntegerOverflow=on  InputSameDT=on
  out_1 : Outport
  wires:
  "[epossp]"/1 -> Switch/3, SampHold?/1(Input)
  Sign/1 -> Switch/2, SampHold?/2(S/H?)
  Gain _/1 -> Sum/1
  SampHold?/1(output) -> Sum/2
  Sum/1 -> Switch/1
  "[pgout]"/1 -> Abs/1, Gain _/1
  Switch/1 -> out_1/1
  Abs/1 -> Sign/1

== system CNcs7/CN/LMLN  03/03/01/IM CN-LMLN/NI Control/Boolify ==
  In1 : Inport  Port=1  LatchInput=off
  Abs2 : Abs  SaturateOnIntegerOverflow=on
  direction1 : Signum
  Out1 : Outport
  wires:
  Abs2/1 -> direction1/1
  In1/1 -> Abs2/1
  direction1/1 -> Out1/1

== system CNcs7/CN/LMLN  03/03/01/IM CN-LMLN/NI Control/Boolify1 ==
  In1 : Inport  Port=1  LatchInput=off
  Abs2 : Abs  SaturateOnIntegerOverflow=on
  direction1 : Signum
  Out1 : Outport
  wires:
  direction1/1 -> Out1/1
  In1/1 -> Abs2/1
  Abs2/1 -> direction1/1

== system CNcs7/CN/LMLN  03/03/01/IM CN-LMLN/NI Control/Boolify2 ==
  In1 : Inport  Port=1  LatchInput=off
  Abs2 : Abs  SaturateOnIntegerOverflow=on
  direction1 : Signum
  Out1 : Outport
  wires:
  Abs2/1 -> direction1/1
  In1/1 -> Abs2/1
  direction1/1 -> Out1/1

== system CNcs7/CN/LMLN  03/03/01/IM CN-LMLN/NI Control/Boolify3 ==
  In1 : Inport  Port=1  LatchInput=off
  Abs2 : Abs  SaturateOnIntegerOverflow=on
  direction1 : Signum
  Out1 : Outport
  wires:
  direction1/1 -> Out1/1
  In1/1 -> Abs2/1
  Abs2/1 -> direction1/1

== system CNcs7/CN/LMLN  03/03/01/IM CN-LMLN/NI Control/DZ .5 ==
  note: We just output zero when the dead zone is in effect, and leave the
      |  output alone the rest of the time.
  note: This block is a better implementation of a dead zone than  the
      | block supplied by SIMULINK, because here we don't _subtract_
      | the dead zone from the rest of output.
  in_1 : Inport  Port=1  LatchInput=off
  Abs : Abs  Orientation=down  SaturateOnIntegerOverflow=on
  Relational Operator : RelationalOperator  InputSameDT=on
  Switch6 : Switch  Threshold=.5  SaturateOnIntegerOverflow=on  InputSameDT=on
  dead zone : Constant  Orientation=up  Value=.5
  pos (deg) criterion1 : Constant  Orientation=left  Value=0
  out_1 : Outport
  wires:
  Relational Operator/1 -> Switch6/2
  dead zone/1 -> Relational Operator/2
  pos (deg) criterion1/1 -> Switch6/3
  Abs/1 -> Relational Operator/1
  in_1/1 -> Switch6/1, Abs/1
  Switch6/1 -> out_1/1

== system CNcs7/CN/LMLN  03/03/01/IM CN-LMLN/NI Control/Zero-Cross ==
  note: Zero Cross Detect
  "[epr]" : Inport  Port=1  LatchInput=off
  Relational Operator : RelationalOperator  Operator=~=  InputSameDT=on
  Sign2 : Signum
  loop breaker1 : Memory
  "[epneq]" : Outport
  wires:
  Relational Operator/1 -> "[epneq]"/1
  loop breaker1/1 -> Relational Operator/2
  "[epr]"/1 -> Sign2/1
  Sign2/1 -> Relational Operator/1, loop breaker1/1

== system CNcs7/CN/LMLN  03/03/01/IM CN-LMLN/NI Control/leading edge detect ==
  note: leading edge detection
  in_1 : Inport  Port=1  LatchInput=off
  Abs : Abs  SaturateOnIntegerOverflow=on
  Derivative : Derivative
  Relational Operator : RelationalOperator  Operator===  InputSameDT=on
  Sign : Signum
  Threshold 1 : Constant
  out_1 : Outport
  wires:
  in_1/1 -> Abs/1
  Relational Operator/1 -> out_1/1
  Threshold 1/1 -> Relational Operator/2
  Sign/1 -> Relational Operator/1
  Derivative/1 -> Sign/1
  Abs/1 -> Derivative/1

== system CNcs7/CN/LMLN  03/03/01/IM CN-LMLN/NI Control/leading edge detect1 ==
  note: leading edge detection
  in_1 : Inport  Port=1  LatchInput=off
  Abs : Abs  SaturateOnIntegerOverflow=on
  Derivative : Derivative
  Relational Operator : RelationalOperator  Operator===  InputSameDT=on
  Sign : Signum
  Threshold 1 : Constant
  out_1 : Outport
  wires:
  Abs/1 -> Derivative/1
  Derivative/1 -> Sign/1
  Sign/1 -> Relational Operator/1
  Threshold 1/1 -> Relational Operator/2
  Relational Operator/1 -> out_1/1
  in_1/1 -> Abs/1

== system CNcs7/CN/LMLN  03/03/01/IM CN-LMLN/NI Control/trailing edge detect ==
  note: It is also possible to remove the SIGNUM function
      | and the '==', and replace them with a simple
      | switch with a threshold of (say) 150 or so.
  note: trailing edge detection
  in_1 : Inport  Port=1  LatchInput=off
  Abs : Abs  SaturateOnIntegerOverflow=on
  Derivative : Derivative
  Relational Operator : RelationalOperator  Operator===  InputSameDT=on
  Sign : Signum
  Threshold 1 : Constant  Value=-1
  out_1 : Outport
  wires:
  Abs/1 -> Derivative/1
  Derivative/1 -> Sign/1
  Sign/1 -> Relational Operator/1
  Threshold 1/1 -> Relational Operator/2
  Relational Operator/1 -> out_1/1
  in_1/1 -> Abs/1

== system CNcs7/CN/LMLN  03/03/01/IM CN-LMLN/Sacc Blank/event timer1 ==
  note: In 2) Subsequent events DO NOT reset the counter; it only resets when it
      | reaches zero
  note: 2) A new event (leading or trailing edge) is detected. -- Only case 1)
  note: 1) The count reaches its limit (set in "timer value") -- Both case 1) and 2)
  note: In 1), Any event (leading or trailing edge) will reset the counter so that it
      | counts down from the end trailing edge) of that event.
  note: It has TWO modes: 1) Event resettable and 2) Event Non-resettable
  note: The real trick here is understanding how to reload the countdown.
      | It resets if either of two conditions is met:
  note: The "OR" gate allows either of these conditions to reset the circuit.  The delay before the
      | "S" input of the flip-flop prevents both "S" and "R" from being set simultaneously, because
      | this would put the flip-flop in an undefined state.
  note: Therefore, an event first RESETS and then SETS the flip-flop.
  note: (Init input: 0)
  note: (FF init state: Q=0)
  note: (Init input: 0)
  note: This block is an RESETTABLE EVENT TIMER.  It outputs a spike of unit height xx milliseconds
      | (set by "timer value") after it detects an event ( i.e a TRAILING edge which represents the end of a
      |  saccadic pulse)
  note: Resettable
      | Event Timer
  _PG : Inport  Port=1  LatchInput=off
  _timer value (port) : Inport  Port=2  LatchInput=off
  1 msec : TransportDelay  DelayTime=.001
  Clock : Clock
      settings: Decimation=10
  Latch1 : simulink_extras/Flip Flops/S-R Flip-Flop  initial_condition=0
  Logical Operator : Logic  Operator=OR  Inputs=3
  Logical Operator1 : Logic
  Logical Operator2 : Logic
  Relational Operator : RelationalOperator  InputSameDT=on
  SampHold?1 : Subsystem
      mask Display: disp('S&H\n(S=L)\n(H=H)')
  Sum : Sum  Inputs=+-  SaturateOnIntegerOverflow=on  InputSameDT=on
  event resettable? : Constant  Orientation=up
  leading edge detect : Subsystem
      mask Display: disp('Leading\nEdge Det')
  loop breaker : Memory  Orientation=left
  trailing edge detect : Subsystem
      mask Display: disp('Trailing\nEdge Det')
  out_1 : Outport
  wires:
  event resettable?/1 -> Logical Operator1/2, Logical Operator2/2
  leading edge detect/1(out_1) -> Logical Operator2/1
  Logical Operator2/1 -> Logical Operator/2
  trailing edge detect/1(out_1) -> 1 msec/1, Logical Operator1/1
  Logical Operator1/1 -> Logical Operator/1
  loop breaker/1 -> Logical Operator/3
  Latch1/1 -> SampHold?1/2(S/H?)
  Sum/1 -> Relational Operator/1
  Clock/1 -> SampHold?1/1(Input), Sum/1
  _PG/1 -> leading edge detect/1(in_1), trailing edge detect/1(in_1)
  Relational Operator/1 -> out_1/1, loop breaker/1
  SampHold?1/1(output) -> Sum/2
  Logical Operator/1 -> Latch1/2
  1 msec/1 -> Latch1/1
  _timer value (port)/1 -> Relational Operator/2
